simulink model "ramps"  (R2018a)
settings: Solver=VariableStepAuto  StartTime=0.0  StopTime=ttotal  RelTol=1e-3
libraries: simulink x7
settings Model: Creator=Carlos  LastModifiedBy=Carlos

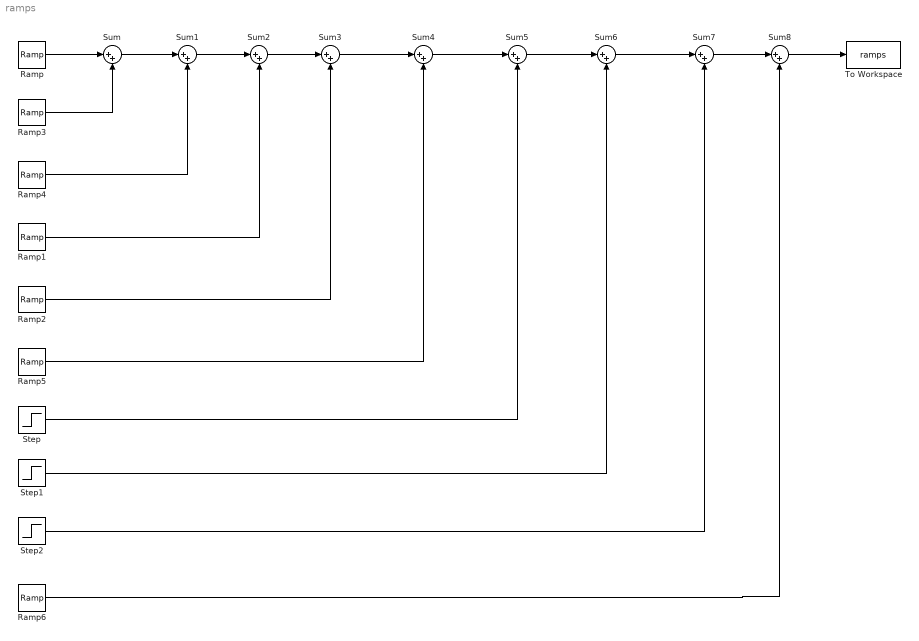
== system ramps ==
  Ramp : simulink/Sources/Ramp  slope=2  start=1  InitialOutput=0
  Ramp1 : simulink/Sources/Ramp  slope=-4  start=5  InitialOutput=0
  Ramp2 : simulink/Sources/Ramp  slope=6  start=7  InitialOutput=0
  Ramp3 : simulink/Sources/Ramp  slope=-2  start=2  InitialOutput=0
  Ramp4 : simulink/Sources/Ramp  slope=4  start=4  InitialOutput=0
  Ramp5 : simulink/Sources/Ramp  slope=-6  start=8  InitialOutput=0
  Ramp6 : simulink/Sources/Ramp  slope=2  start=10  InitialOutput=0
  Step : Step  Time=2  After=-2  SampleTime=0
  Step1 : Step  Time=5  After=-4  SampleTime=0
  Step2 : Step  Time=8  After=-6  SampleTime=0
  Sum{,1..8} (9 alike) : Sum  Inputs=|++
  To Workspace : ToWorkspace  VariableName=ramps  SampleTime=-1
  wires:
  Ramp/1 -> Sum/1
  Sum/1 -> Sum1/1
  Sum1/1 -> Sum2/1
  Sum2/1 -> Sum3/1
  Ramp3/1 -> Sum/2
  Ramp4/1 -> Sum1/2
  Ramp1/1 -> Sum2/2
  Ramp2/1 -> Sum3/2
  Sum6/1 -> Sum7/1
  Sum5/1 -> Sum6/1
  Sum4/1 -> Sum5/1
  Sum3/1 -> Sum4/1
  Ramp5/1 -> Sum4/2
  Step/1 -> Sum5/2
  Step1/1 -> Sum6/2
  Step2/1 -> Sum7/2
  Ramp6/1 -> Sum8/2
  Sum8/1 -> To Workspace/1
  Sum7/1 -> Sum8/1
